simulink model "limbControl1"  (R2018b)
settings: Solver=FixedStepAuto  StartTime=0.0  StopTime=248  FixedStep=Ts  RelTol=1e-3
InitFcn:
  | init
values from neighbouring files (symbols this model uses):
  B1 = 0    [init.m]
  B2 = 0.01    [init.m]
  B3 = 1    [init.m]
  g = 10    [init.m]
  J = 1    [init.m]
  K1 = 0    [init.m]
  K2 = 0.01    [init.m]
  K3 = 0    [init.m]
  l = 0.4    [init.m]
  m = 1    [gpcData.mat]    (also in init.m = 3; limb.m; mountVectorU.m = size(U,1))
  Td = 0    [init.m]
undefined symbols (not defined in the file or in its folder): gpcOnline
libraries: simulink x1
settings Model: Creator=hhhhh  LastModifiedBy=hhhhh

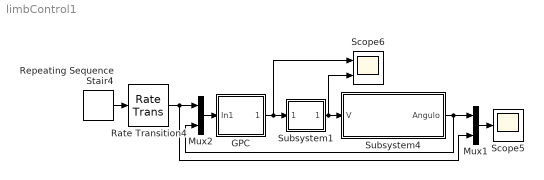
== system limbControl1 ==
  GPC : Subsystem
  Mux1 : Mux  Inputs=2
  Mux2 : Mux  Inputs=2
  Rate Transition4 : RateTransition
  Repeating Sequence Stair4 : simulink/Sources/Repeating Sequence Stair  OutValues="1.3*[0\t0.0523359562429438\t0.104528463267653\t0.156434465040231\t0.207911690817759\t0.258819045102521\t0.309016994374947\t0.358367949545300\t0.406736643075800\t0.453990499739547\t0.500000000000000\t0.544639035015027\t0.587785252292473\t0.629320391049837\t0.669130606358858\t0.707106781186548\t0.743144825477394\t0.777145961456971\t0.809016994374948\t0.838670567945424\t0.866025403784439\t0.891006524188368\t0.913545457642601\t0.933580426497202\t0.951056516295154\t0.965925826289068\t0.978147600733806\t0.987688340595138\t0.994521895368273\t0.998629534754574\t1\t0.998629534754574\t0.994521895368273\t0.987688340595138\t0.978147600733806\t0.965925826289068\t0.951056516295154\t0.933580426497202\t0.913545457642601\t0.891006524188368\t0.866025403784439\t0.838670567945424\t0.809016994374948\t0.777145961456971\t0.743144825477394\t0.707106781186548\t0.669130606358858\t0.629320391049837\t0.587785252292473\t0.544639035015027\t0.500000000000000\t0.453990499739547\t0.406736643075800\t0.358367949545300\t0.309016994374948\t0.258819045102521\t0.207911690817759\t0.156434465040231\t0.104528463267654\t0.0523359562429438].'"  tsamp=4  OutMin=[]  OutMax=[]  OutDataTypeStr=double  OutputDataTypeScalingMode=double  OutDataType=fixdt(0,8)  ConRadixGroup=Best Precision: Vector-wise  OutScaling=2^-12
  Scope5 : Scope
  Scope6 : Scope  NumInputPorts=2
  Subsystem1 : Subsystem
  Subsystem4 : Subsystem
  wires:
  Subsystem1/1(Out1) -> Subsystem4/1(V), Scope6/2
  Mux1/1 -> Scope5/1
  Repeating Sequence Stair4/1 -> Rate Transition4/1
  Subsystem4/1(Angulo) -> Mux2/2, Mux1/1
  Rate Transition4/1 -> Mux2/1, Mux1/2
  GPC/1(Out1) -> Scope6/1, Subsystem1/1(In1)
  Mux2/1 -> GPC/1(In1)

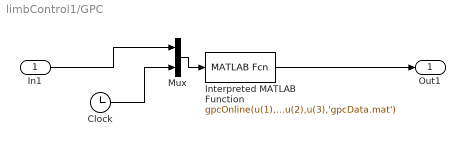
== system limbControl1/GPC ==
  In1 : Inport
  Clock : Clock
  Interpreted MATLAB Function : MATLABFcn  MATLABFcn=gpcOnline(u(1),u(2),u(3),'gpcData.mat')  OutputDimensions=1
  Mux : Mux  Inputs=2
  Out1 : Outport
  wires:
  Interpreted MATLAB Function/1 -> Out1/1
  In1/1 -> Mux/1
  Mux/1 -> Interpreted MATLAB Function/1
  Clock/1 -> Mux/2

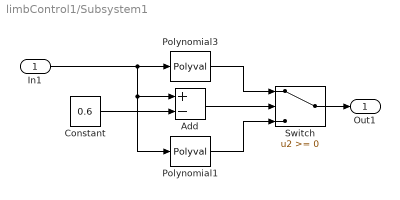
== system limbControl1/Subsystem1 ==
  In1 : Inport
  Add : Sum  Inputs=+-
  Constant : Constant  Value=0.6
  Polynomial1 : Polyval  Coefs=|
      | [0
      | 0
      | 0
      | 4.96473696106646
      | 0
      | 1.22506777764656
      | 11.8762695363768
      | 0]
  Polynomial3 : Polyval  Coefs=|
      | [1334.93659745298
      | -7873.77408130260
      | 19679.6581173489
      | -26904.1335294621
      | 21674.5719980287
      | -10255.6450049827
      | 2645.19572957251
      | -282.136494548769]
  Switch : Switch
  Out1 : Outport
  wires:
  Switch/1 -> Out1/1
  In1/1 -> Add/1, Polynomial1/1, Polynomial3/1
  Constant/1 -> Add/2
  Add/1 -> Switch/2
  Polynomial3/1 -> Switch/1
  Polynomial1/1 -> Switch/3

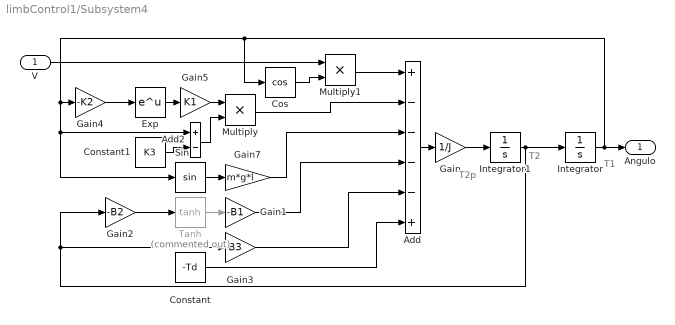
== system limbControl1/Subsystem4 ==
  note: T1
  note: T2p
  note: T2
  V : Inport
  Add : Sum  Inputs=+----+
  Add2 : Sum  Inputs=+-
  Constant : Constant  Value=-Td
  Constant1 : Constant  Value=K3
  Cos : Trigonometry  Operator=cos
  Exp : Math  SaturateOnIntegerOverflow=on
  Gain : Gain  Gain=1/J
  Gain1 : Gain  Gain=-B1
  Gain2 : Gain  Gain=-B2
  Gain3 : Gain  Gain=B3
  Gain4 : Gain  Gain=-K2
  Gain5 : Gain  Gain=K1
  Gain7 : Gain  Gain=m*g*l
  Integrator : Integrator
  Integrator1 : Integrator
  Multiply : Product
  Multiply1 : Product
  Sin : Trigonometry
  Tanh : Trigonometry  Commented=on  Operator=tanh
  Angulo : Outport
  wires:
  Integrator/1 -> Gain4/1, Add2/1, Sin/1, Cos/1, Angulo/1
  Gain2/1 -> Tanh/1
  Integrator1/1 -> Gain2/1, Gain3/1, Integrator/1
  Exp/1 -> Gain5/1
  Gain7/1 -> Add/3
  Sin/1 -> Gain7/1
  V/1 -> Multiply1/1
  Add2/1 -> Multiply/2
  Multiply1/1 -> Add/1
  Gain4/1 -> Exp/1
  Multiply/1 -> Add/2
  Tanh/1 -> Gain1/1
  Add/1 -> Gain/1
  Cos/1 -> Multiply1/2
  Gain3/1 -> Add/5
  Constant/1 -> Add/6
  Gain1/1 -> Add/4
  Gain5/1 -> Multiply/1
  Gain/1 -> Integrator1/1
  Constant1/1 -> Add2/2
